simulink model "Hardware_testng_simulink_both"  (R2024b)
settings: Solver=ode1  StartTime=0.0  StopTime=15  FixedStep=0.005  RelTol=1e-3  EnableMultiTasking=on
undefined symbols (not defined in the file or in its folder): DiscIntNeverNeededParam, initialPose, maxAngularAcc, maxAngularVel, maxLinearAcc, maxLinearVel, poseTol, Ts, wps1
libraries: simulink_extras x12, stmnucleolib x12, simulink x4, hdlsllib x1, embmathops x1, robotcorelib x1
(part 2 of 2)

== matlab function Hardware_testng_simulink_both/Waypoint Trajectory/3D Waypoint for Auto ==
  settings: updateMethod=DISCRETE
  data: genAcc output size=[4,1]; Ts output size=[1,1]; t input; departTime input; departPose input; targetPose input; maxVel input; maxAcc input
 function [genAcc,Ts] = fcn(t,departTime,departPose,targetPose,maxVel,maxAcc)
%#codegen

persistent  t1 prevVel
if isempty(t1)
    t1 = 0; prevVel = [0;0;0;0];
end

Ts = t-t1;
t1 = t;
maxLinearAcc    = abs(maxAcc(1));
maxAngularAcc   = abs(maxAcc(2));
maxLinearVel    = abs(maxVel(1));
maxAngularVel   = abs(maxVel(2));
if maxLinearAcc  == 0, maxLinearAcc  = 1e-5;end
if maxAngularAcc == 0, maxAngularAcc  = 1e-5;end
if maxLinearVel  == 0, maxLinearVel  = 1e-5;end
if maxAngularVel == 0, maxAngularVel = 1e-5;end

dxyz        = targetPose(1:3) - departPose(1:3);
dyaw        = targetPose(4) - departPose(4);
distance    = norm(dxyz);
twoMinDist  = maxLinearVel^2/maxLinearAcc;
distAngle   = abs(dyaw);
twoMinTheta = maxAngularVel^2/maxAngularAcc;

vel = zeros(4,1);
if distance > twoMinDist
    ta  = maxLinearVel/maxLinearAcc;
    tad = (distance - twoMinDist)/maxLinearVel;
    td  = ta + tad;
    te  = ta + td;
    if (t-departTime) < ta
        velxyz = maxLinearAcc*(t-departTime);
    elseif ta <= (t-departTime) && (t-departTime) < td
        velxyz = maxLinearVel;
    elseif td <= (t-departTime) && (t-departTime) < te
        velxyz = -maxLinearAcc*(t-departTime-td) + maxLinearVel;
    else
        velxyz = 0;
    end
else
    tp = sqrt(distance/maxLinearAcc);
    te = 2*tp;
    velp = maxLinearAcc*tp;
    if (t-departTime) < tp
        velxyz = maxLinearAcc*(t-departTime);
    elseif tp <= (t-departTime) && (t-departTime) < te
        velxyz = -maxLinearAcc*(t-departTime-tp)+velp;
    else
        velxyz = 0;
    end
end
if distance ~=0
    vel(1:3) = velxyz*dxyz/distance;
end

if distAngle > twoMinTheta
    ta  = maxAngularVel/maxAngularAcc;                   % acceleration period
    tad = (distAngle-twoMinTheta)/maxAngularVel; % acc to deceleration period
    td  = ta + tad;                  % start deceleration
    te  = ta + td;                   % end deceleration
    if (t-departTime) < ta
        omega = maxAngularAcc*(t-departTime);
    elseif ta <= (t-departTime) && (t-departTime) < td
        omega = maxAngularVel;
    elseif td <= (t-departTime) && (t-departTime) < te
        omega = -maxAngularAcc*(t-departTime-td) + maxAngularVel;
    else
        omega = 0;
    end
else
    tp = sqrt(distAngle/maxAngularAcc);
    te = 2*tp;
    omegap = maxAngularAcc*tp;
    if (t-departTime) < tp
        omega = maxAngularAcc*(t-departTime);
    elseif tp <= (t-departTime) && (t-departTime) <= te
        omega = -maxAngularAcc*(t-departTime-tp)+omegap;
    else
        omega = 0;
    end
end
vel(4) = omega*sign(dyaw);
if abs(Ts)<1e-6
    genAcc = [0;0;0;0];
else
    genAcc = (vel - prevVel)/Ts;
end
prevVel = vel;
%genAcc_row = genAcc';

== matlab function Hardware_testng_simulink_both/Subsystem4/MATLAB Function2 ==
  data: i input; y output; x input; curr_x input
function y = fcn(i, x, curr_x)
persistent total;
if isempty(total)
    total = 495;
end

if x == 0
    y = total;
else
    if i == 1 && curr_x < 550
        total = total + x;
    elseif i == -1 && curr_x > 400
        total = total + x;
    else
        total = total;
    end
    y = total;
end

end

== matlab function Hardware_testng_simulink_both/Sub_En1_3/Subsystem4/MATLAB Function ==
  data: data input; position output; speed output
function [position, speed] = fcn(data)
    %#codegen
    position = zeros(1, 1, 'single');
    speed = zeros(1, 1, 'single');

    if numel(data) >= 8
        position = typecast(data(1:4), 'single');
        speed = typecast(data(5:8), 'single');
    end
end

== matlab function Hardware_testng_simulink_both/Sub_En1_3/Subsystem5/MATLAB Function ==
  data: data input; position output; speed output
function [position, speed] = fcn(data)
    %#codegen
    position = zeros(1, 1, 'single');
    speed = zeros(1, 1, 'single');

    if numel(data) >= 8
        position = typecast(data(1:4), 'single');
        speed = typecast(data(5:8), 'single');
    end
end

== matlab function Hardware_testng_simulink_both/Subsystem4/MATLAB Function3 ==
  data: i input; y output; x input
function y = fcn(i,x)
if i == 1 && x < 0.6
    y = x+0.5;
elseif i == 1 && x == 0.6 && x > 0.6
    x = x;
    y = 0.6;
elseif i == -1 && x > -0.6
    y = x-0.5;
elseif i == -1 && x == -0.6 && x < -0.6
    x = x;
    y = -0.6;
elseif i == 0
    y = 0;
else 
    y = x;

end

end

== matlab function Hardware_testng_simulink_both/Subsystem5/MATLAB Function ==
  data: i input; y output; x input; curr_x input
function y = fcn(i, x, curr_x)
persistent total;
if isempty(total)
    total = 661;
end

if x == 0
    y = total;
else
    if i == 1 && curr_x < 680
        total = total + x;
    elseif i == -1 && curr_x > 351
        total = total + x;
    else
        total = total;
    end
    y = total;
end

end

== matlab function Hardware_testng_simulink_both/Subsystem5/MATLAB Function1 ==
  data: i input; y output; x input
function y = fcn(i,x)
if i == 1 && x < 0.6
    y = x+0.5;
elseif i == 1 && x == 0.6 && x > 0.6
    x = x;
    y = 0.6;
elseif i == -1 && x > -0.6
    y = x-0.5;
elseif i == -1 && x == -0.6 && x < -0.6
    x = x;
    y = -0.6;
elseif i == 0
    y = 0;
else 
    y = x;

end

end

== matlab function Hardware_testng_simulink_both/Subsystem6/MATLAB Function2 ==
  data: i input; y output; x input; curr_x input
function y = fcn(i, x, curr_x)
persistent total;
if isempty(total)
    total = 0;
end

if x == 0
    y = total;
else
    if i == 1 && curr_x < 300
        total = total + x;
    elseif i == -1 && curr_x > -300
        total = total + x;
    elseif i ~= 0 && curr_x > -10 && curr_x <10
        y = 0;
        total = 0;
    else
        total = total;
    end
    y = total;
end

end

== matlab function Hardware_testng_simulink_both/Subsystem6/MATLAB Function3 ==
  data: i input; y output; x input
function y = fcn(i,x)
if i == 1 && x < 0.6
    y = x+0.5;
elseif i == 1 && x == 0.6 && x > 0.6
    x = x;
    y = 0.6;
elseif i == -1 && x > -0.6
    y = x-0.5;
elseif i == -1 && x == -0.6 && x < -0.6
    x = x;
    y = -0.6;
elseif i == 0
    y = 0;
else 
    y = x;

end

end

== matlab function Hardware_testng_simulink_both/Inverse_forward Kinematic/Subsystem/Define Relative angle ==
  settings: updateMethod=DISCRETE
  data: initialPose input; reset_angle input; rawangle input; angle output; status input
function angle = fcn(initialPose, reset_angle, rawangle, status)

% continuousangle is absolute angle
% angle is relative angle

persistent prevPsi2pi jump rawangle_0 set_angle
if isempty(prevPsi2pi)
    prevPsi2pi = 0; jump = 0; rawangle_0 = rawangle; set_angle = 0;
end

if abs(rawangle-prevPsi2pi) >  pi
    if rawangle > 0
        jump = jump - 1;
    else
        jump = jump + 1;
    end
end
if abs(rawangle-prevPsi2pi) >  pi/2 && abs(rawangle-prevPsi2pi) < pi
    if rawangle > 0
        jump = jump - 1/2;
    else
        jump = jump + 1/2;
    end
end

prevPsi2pi = rawangle;

continuousangle = rawangle + jump*2*pi; % continuous value

if (status && ~set_angle), rawangle_0 = continuousangle; set_angle  = 1; end

if reset_angle, rawangle_0 = continuousangle; end

angle = continuousangle - rawangle_0 + initialPose;

== matlab function Hardware_testng_simulink_both/Inverse Kinematic1 ==
  settings: updateMethod=DISCRETE
  data: Px input; q1 output; Py input; Pz input; q2 output; q3 output; q4 output; q5 output; q6 output; R06 input
function [q1, q2, q3, q4, q5, q6] = inverseKinematics(Px, Py, Pz, R06)
    % Define actual geometry parameters (in meters)
%     l1 = 276;        % Length of link 1
%     l2 = 305.94661;  % Length of link 2
%     l3 = 154.46177;  % Length of link 3
%     l4 = 228.74688;  % Length of link 4
%     l5 = 68.15773;   % Length of link 5 (offset)
%     l6 = 41.47212;   % Length of link 6 (end-effector)
%     a  = 82.4965;    % Offset a
%%Old length 
l1=276;
l2=306;
a=79.75;
l3=160;
l4=227;
l5=70;
l6=38;

%     R06=[0    0   1
%          0   -1   0
%          1    0   0];
    % Wrist position calculation
    O6=[Px,Py,Pz]';
    d6=l5+l6;
    OW = O6 - R06*[0;0;d6];
%     r13 = R06(1, 3);
%     r23 = R06(2, 3);
%     r33 = R06(3, 3);

    % Compute wrist position (compensating for the end-effector offset)
%     Pwx = Px - (l5 + l6) * r13;
%     Pwy = Py - (l5 + l6) * r23;
%     Pwz = Pz - (l5 + l6) * r33;
Pwx=OW(1); Pwy=OW(2);Pwz=OW(3);

    % Compute q1 directly from the wrist position
    q1 = atan2(Pwy, Pwx);

    % Convert wrist position to cylindrical coordinates
    r = sqrt(Pwx^2 + Pwy^2);
    %new code 
    h= Pwz-l1;
    % my code: h = Pwz - l1;

    % Intermediate calculations for q2 and q3
    s = sqrt(h^2 + r^2);
    alp = atan(h/r );
    w3 = l3 + l4;
    k3 = sqrt(a^2 + w3^2);
    %phi2
    beta = acos((l2^2 + s^2 - k3^2) / (2 * l2 * s));
   %gamma or phi3
    gamma = acos(( l2^2+k3^2-s^2) / (2 * l2 * k3));
    Phi = atan(w3/a);
    

    % Target angles for q2 and q3
    q2 = (-alp -beta+pi/2);
    q3 = (pi-gamma - Phi);
%     q3= -gamma-pi/2;

    % Compute R0_3 from q1, q2, q3
    R03 = [cos(q1)*cos(q2 + q3), -cos(q1)*sin(q2 + q3), -sin(q1);
           sin(q1)*cos(q2 + q3), -sin(q1)*sin(q2 + q3),  cos(q1);
           -sin(q2 + q3)       , -cos(q2 + q3)        , 0 ];
    R03t=transpose(R03);

    % Compute R3_6 from the known R0_3 and R0_6
    R3_6 = R03t* R06;

    % Extract elements from R3_6 for calculating q4, q5, q6
    s5c4 = -R3_6(1, 3);
    c5   = R3_6(2, 3);
    s5s4 = R3_6(3, 3);
    s5c6 = R3_6(2, 1);
    s5s6 = -R3_6(2, 2);

    % Joint angle q5
%     q5m = atan2(-sqrt(1 - c5^2), c5);
      q5p = atan2(-sqrt(1-c5^2),c5);
% q5p=asin(c5);
% 
%     % Joint angles q4 and q6 based on the sign of q5
%     if q5m > q5p
%        q5=q5m;
%     q5=q5p;
%        q4 = atan2(s5s4  , s5c4);
%        q6 = atan2(s5s6, s5c6);
%     else    
      q5=q5p;
        q4 = atan2(-s5s4, s5c4);
        q6 = atan2(-s5s6, -s5c6);
    
%     end
end

== matlab function Hardware_testng_simulink_both/Inverse_forward Kinematic/Subsystem14/Define Relative angle ==
  settings: updateMethod=DISCRETE
  data: initialPose input; reset_angle input; rawangle input; angle output; status input
function angle = fcn(initialPose, reset_angle, rawangle, status)

% continuousangle is absolute angle
% angle is relative angle

persistent prevPsi2pi jump rawangle_0 set_angle
if isempty(prevPsi2pi)
    prevPsi2pi = 0; jump = 0; rawangle_0 = rawangle; set_angle = 0;
end

if abs(rawangle-prevPsi2pi) >  pi
    if rawangle > 0
        jump = jump - 1;
    else
        jump = jump + 1;
    end
end
if abs(rawangle-prevPsi2pi) >  pi/2 && abs(rawangle-prevPsi2pi) < pi
    if rawangle > 0
        jump = jump - 1/2;
    else
        jump = jump + 1/2;
    end
end

prevPsi2pi = rawangle;

continuousangle = rawangle + jump*2*pi; % continuous value

if (status && ~set_angle), rawangle_0 = continuousangle; set_angle  = 1; end

if reset_angle, rawangle_0 = continuousangle; end

angle = continuousangle - rawangle_0 + initialPose;

== matlab function Hardware_testng_simulink_both/Inverse_forward Kinematic/Subsystem15/Define Relative angle ==
  settings: updateMethod=DISCRETE
  data: initialPose input; reset_angle input; rawangle input; angle output; status input
function angle = fcn(initialPose, reset_angle, rawangle, status)

% continuousangle is absolute angle
% angle is relative angle

persistent prevPsi2pi jump rawangle_0 set_angle
if isempty(prevPsi2pi)
    prevPsi2pi = 0; jump = 0; rawangle_0 = rawangle; set_angle = 0;
end

if abs(rawangle-prevPsi2pi) >  pi
    if rawangle > 0
        jump = jump - 1;
    else
        jump = jump + 1;
    end
end
if abs(rawangle-prevPsi2pi) >  pi/2 && abs(rawangle-prevPsi2pi) < pi
    if rawangle > 0
        jump = jump - 1/2;
    else
        jump = jump + 1/2;
    end
end

prevPsi2pi = rawangle;

continuousangle = rawangle + jump*2*pi; % continuous value

if (status && ~set_angle), rawangle_0 = continuousangle; set_angle  = 1; end

if reset_angle, rawangle_0 = continuousangle; end

angle = continuousangle - rawangle_0 + initialPose;

== matlab function Hardware_testng_simulink_both/Inverse_forward Kinematic/Subsystem16/Define Relative angle ==
  settings: updateMethod=DISCRETE
  data: initialPose input; reset_angle input; rawangle input; angle output; status input
function angle = fcn(initialPose, reset_angle, rawangle, status)

% continuousangle is absolute angle
% angle is relative angle

persistent prevPsi2pi jump rawangle_0 set_angle
if isempty(prevPsi2pi)
    prevPsi2pi = 0; jump = 0; rawangle_0 = rawangle; set_angle = 0;
end

if abs(rawangle-prevPsi2pi) >  pi
    if rawangle > 0
        jump = jump - 1;
    else
        jump = jump + 1;
    end
end
if abs(rawangle-prevPsi2pi) >  pi/2 && abs(rawangle-prevPsi2pi) < pi
    if rawangle > 0
        jump = jump - 1/2;
    else
        jump = jump + 1/2;
    end
end

prevPsi2pi = rawangle;

continuousangle = rawangle + jump*2*pi; % continuous value

if (status && ~set_angle), rawangle_0 = continuousangle; set_angle  = 1; end

if reset_angle, rawangle_0 = continuousangle; end

angle = continuousangle - rawangle_0 + initialPose;

== matlab function Hardware_testng_simulink_both/Subsystem13/Define Relative angle1 ==
  settings: updateMethod=DISCRETE
  data: initialPose input; reset_angle input; rawangle input; angle output; status input
function angle = fcn(initialPose, reset_angle, rawangle, status)

% continuousangle is absolute angle
% angle is relative angle

persistent prevPsi2pi jump rawangle_0 set_angle
if isempty(prevPsi2pi)
    prevPsi2pi = 0; jump = 0; rawangle_0 = rawangle; set_angle = 0;
end

if abs(rawangle-prevPsi2pi) >  pi
    if rawangle > 0
        jump = jump - 1;
    else
        jump = jump + 1;
    end
end
prevPsi2pi = rawangle;

continuousangle = rawangle + jump*2*pi; % continuous value

if (status && ~set_angle), rawangle_0 = continuousangle; set_angle  = 1; end

if reset_angle, rawangle_0 = continuousangle; end

angle = continuousangle - rawangle_0 + initialPose;

== matlab function Hardware_testng_simulink_both/Waypoint Trajectory/1st Order Filter ==
  data: Y_dot input; Y input; X input; Y_ddot output
function Y_ddot = fcn(Y_dot,Y,X)

Y_ddot = zeros(4,1);
zeta = 1;
wn = 2*pi*1;

Y_ddot(1) = (-wn*wn*Y(1) - 2*zeta*wn*Y_dot(1) + wn*wn*X(1));
Y_ddot(2) = (-wn*wn*Y(2) - 2*zeta*wn*Y_dot(2) + wn*wn*X(2));
Y_ddot(3) = (-wn*wn*Y(3) - 2*zeta*wn*Y_dot(3) + wn*wn*X(3));
Y_ddot(4) = (-wn*wn*Y(4) - 2*zeta*wn*Y_dot(4) + wn*wn*X(4));
